simulink model "zynqRadioWLAN80211BeaconRxFPGAAD9361AD9364RetargetSL"  (R2016a)
settings: Solver=FixedStepDiscrete  SolverMode=SingleTasking  StartTime=0.0  StopTime=inf  RelTol=1e-3
PreLoadFcn:
  | load('commwlan80211BusTypes')
  | openMPDUGUI = true;
PostLoadFcn:
  | zynqRadioWLAN80211BeaconRxFPGAAD9361AD9364SL_params('init')
  | zynqRadioWLAN80211BeaconRxFPGAAD9361AD9364SL_params('retarget_scope')
InitFcn:
  | load('commwlan80211BusTypes')
  | openMPDUGUI = true;
  | mpduFigPos= [ 100 100 400 500];
model workspace: external: MAT-File (data not in the file)
undefined symbols (not defined in the file or in its folder): F, p80211
libraries: commutil2 x3, hdlsllib x3, commwlan80211BeaconLib x2, commdigbbndpm3 x1, commsequence2 x1, simulink x1, commcrc2 x1, sdrzblksprivate x1, zc706fmc234_lib x1
CloseFcn:
  | clear BeaconFrameBodyType BeaconMPDUType CapabilityType FrameCtrlType InfoElementType MPDUHeaderType p80211 commwlan80211TxFilt rcvd openMPDUGUI mpduFigPos p80211hdl Hd
  | hFig = findall(0, 'Type', 'figure', 'Name', '802.11 Beacon Frame');
  | if ishghandle(hFig)
  | close(hFig);
  | end
  | clear hFig
  | if (exist('ans')==1) && (iscell(ans) && (numel(ans) == 0))
  | clear ans
  | end
Description:
  | IEEE 802.11 WLAN Beacon Frame Receiver for Captured Data
  | 
  | This example shows how to process a captured beacon frame and display the
  | frame information.
settings Model: ModifiedByFormat=The MathWorks Inc.  SimulationMode=accelerator  ExtModeTrigDuration=100  Creator=The MathWorks, Inc.  LastModifiedBy=The MathWorks Inc.
settings DataIOCC: LimitDataPoints=on  SaveFormat=Array  SaveOutput=off  SignalLogging=off  DSMLogging=off  StateSaveName=tmp_raccel_xout
settings OptimizationCC: BlockReduction=off  ConditionallyExecuteInputs=off  DefaultParameterBehavior=Inlined  InlineInvariantSignals=on  ExpressionDepthLimit=2147483647  EfficientMapNaN2IntZero=off
settings DebuggingCC: ReadBeforeWriteMsg=DisableAll  WriteAfterWriteMsg=DisableAll  WriteAfterReadMsg=DisableAll  AlgebraicLoopMsg=error  UnderspecifiedInitializationDetection=Classic  MergeDetectMultiDrivingBlocksExec=none  SolverPrmCheckMsg=warning  InheritedTsInSrcMsg=none  SingleTaskRateTransMsg=error  IntegerOverflowMsg=none  ParameterDowncastMsg=none  ParameterOverflowMsg=none  ParameterPrecisionLossMsg=none  ParameterTunabilityLossMsg=none  UniqueDataStoreMsg=error  AllowSymbolicDim=off  ModelReferenceDataLoggingMessage=none  StateNameClashWarn=warning  IntegerSaturationMsg=none
settings HardwareCC: ProdBitPerPointer=32  ProdLargestAtomicFloat=None  ProdIntDivRoundTo=Undefined  ProdEndianess=Unspecified  ProdWordSize=32  ProdHWDeviceType=ASIC/FPGA->ASIC/FPGA  TargetBitPerPointer=64  TargetLongLongMode=on  TargetIntDivRoundTo=Zero  TargetEndianess=LittleEndian  TargetWordSize=64  TargetHWDeviceType=MATLAB Host  ProdEqTarget=off
settings ModelReferenceCC: PropagateSignalLabelsOutOfModel=off
settings RTWCC: SystemTargetFile=raccel.tlc  TemplateMakefile=raccel_default_tmf  RTWVerbose=off  RTWUseSimCustomCode=on
settings CodeAppCC: GenerateComments=off  MaxIdLength=128  MangleLength=10  SimulinkBlockComments=off
settings RaccelTargetCC: ERTMultiwordTypeDef=System defined  ERTMultiwordLength=256  ParMdlRefBuildCompliant=off  GeneratePreprocessorConditionals=Disable all  ERTFirstTimeCompliant=off  MultiInstanceERTCode=off  ENABLE_SLEXEC_SSBRIDGE=0  RTWCAPISignals=off  RTWCAPIParams=off
settings ConfigComp: CovModelRefEnable=Off  CovSFcnEnable=off

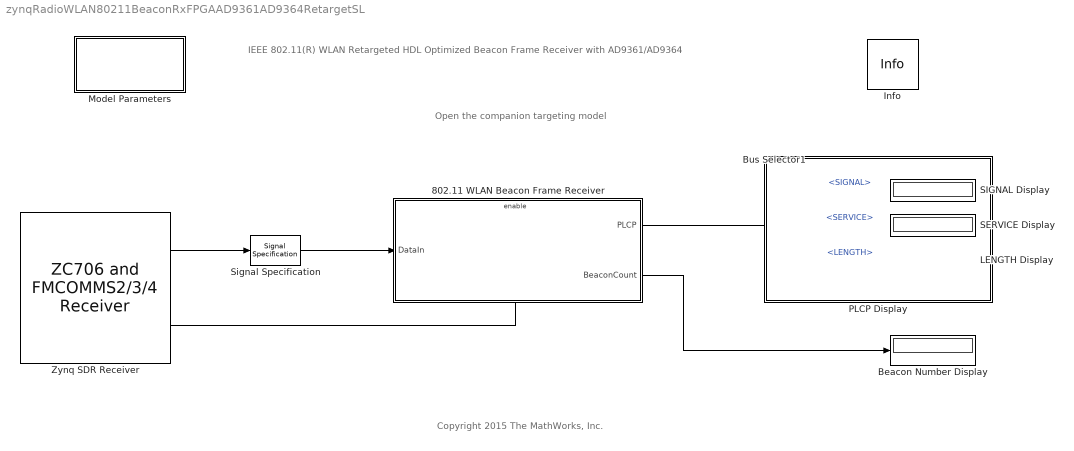
== system zynqRadioWLAN80211BeaconRxFPGAAD9361AD9364RetargetSL ==
  note: IEEE 802.11(R) WLAN
      | Retargeted HDL Optimized Beacon Frame Receiver with AD9361/AD9364
  note: Copyright 2015 The MathWorks, Inc.
  note: Open the companion targeting model
  802.11 WLAN Beacon Frame Receiver : Subsystem
  Beacon Number Display : Display
  Bus Selector1 : BusSelector  OutputSignals=SIGNAL,SERVICE,LENGTH
  Info : sdrzblksprivate/Info  SystemSampleTime=-1
  LENGTH Display : Display
  Model Parameters : Subsystem  mask(Model Parameters){chanNum=1, rfGain=30, rfFreqOffset=0}
      mask prompts: chanNum "Channel number"; rfGain "RF board gain:"; rfFreqOffset "RF center frequency offset:"
      mask help:
      | Choose 802.11 receiver parameters.
      |
      | You can select channel number for the 802.11 signals. You can set the AGC parameters and samples per chip used in the receiver. You can also set the synchronization threshold value to determine the correlation threshold used to declare the presence of an 802.11 packet.
      mask init:
      | zynqRadioWLAN80211BeaconRxFPGAAD9361AD9364SL_params('init', ...
      |     'ChannelNumber',   chanNum, ...
      |     'RadioGain',       rfGain, ...
      |     'RadioFreqOffset', rfFreqOffset ...
      |     );
      mask TypeOptions chanNum: 1 | 2 | 3 | 4 | 5 | 6 | 7 | 8 | 9 | 10 | 11
      mask Display: disp('Model\nParameters')
  PLCP Display : Subsystem
      mask Display: disp('')
  SERVICE Display : Display
      settings: Format=hex (Stored Integer)
  SIGNAL Display : Display
      settings: Format=hex (Stored Integer)
  Signal Specification : SignalSpecification  SampleTime=p80211.RadioFrameLength/p80211.RadioBasebandRate
  Zynq SDR Receiver : zc706fmc234_lib/ZC706 and  FMCOMMS2//3//4  Receiver  IPAddress=192.168.3.2  CenterFrequencySource=Dialog  CenterFrequency=2.412e9+(p80211.ChannelNumber-1)*5e6+p80211.RadioFreqOffset  GainSource=Dialog  Gain=p80211.RadioGain  ChannelMapping=1  BasebandSampleRate=p80211.RadioBasebandRate  EnableBurstMode=on  NumFramesInBurst=p80211.RadioNumFramesInBurst  OutputDataType=int16  SamplesPerFrame=p80211.RadioFrameLength  LostSamplesOutputPort=off  RSSIOutputPort=off  DMATimeoutValue=1  blockMode=Normal  EnableQuadratureTracking=on  EnableRFDCTracking=on  EnableBasebandDCTracking=on  BypassUserLogic=off  ShowAdvancedProperties=on  ShowInternalProperties=off  subDeviceList=zynqReceiver  sdrExecutionMode=HW  dataUDPPort=-1  ctrlUDPPort=-1  SourceSelect=RF data  SourceConfiguration1=1023  FIRCoefficientSize=[ 128; 128 ]  FIRCoefficients=[ 111, -87, 147, -127, -18, -286, -312, -555, -601, -722, -642, -555, -303, -66, 221, 393, 488, 403, 219, -74, -343, -550, -582, -450, -146, 221, 569, 759, 735, 463, 20, -487, -885, -1048, -883, -418, 243, 897, 1340, 1394, 1002, 228, -715, -1549, -1980, -1819, -1028, 217, 1583, 2635, 2980, 2377, 853, -1275, -3435, -4926, -5080, -3454, 40, 5065, 10903, 16581, 21085, 23573, 23573, 21085, 16581, 10903, 5065, 40, -3454, -5080, -4926, -3435, -1275, 853, 2377, 2980, 2635, 1583, 217, -1028, -1819, -1980, -1549, -715, 228, 1002, 1394, 1340, 897, 243, -418, -883, -1048, -885, -487, 20, 463, 735, 759, 569, 221, -146, -450, -582, -550, -343, -74, 219, 403, 488, 393, 221, -66, -303, -555, -642, -722, -601, -555, -312, -286, -18, -127, 147, -87, 111; 382, -200, 711, -41, 645, 36, 346, -194, -119, -543, -472, -646, -404, -312, 45, 197, 413, 346, 241, -93, -373, -680, -755, -689, -356, 51, 515, 795, 870, 609, 136, -488, -1009, -1303, -1191, -712, 69, 885, 1516, 1692, 1336, 468, -662, -1740, -2378, -2329, -1494, -55, 1620, 2995, 3584, 3045, 1368, -1121, -3755, -5708, -6156, -4542, -710, 4969, 11669, 18243, 23486, 26391, 26391, 23486, 18243, 11669, 4969, -710, -4542, -6156, -5708, -3755, -1121, 1368, 3045, 3584, 2995, 1620, -55, -1494, -2329, -2378, -1740, -662, 468, 1336, 1692, 1516, 885, 69, -712, -1191, -1303, -1009, -488, 136, 609, 870, 795, 515, 51, -356, -689, -755, -680, -373, -93, 241, 346, 413, 197, 45, -312, -404, -646, -472, -543, -119, -194, 346, 36, 645, -41, 711, -200, 382 ]  FIRGain=[ 0; -12 ]  FIRDecimInterpFactor=[ 4; 4 ]  AnalogFilterCutoff=[ 2560000; 2560000 ]  FilterPathRates=[ 737280000, 184320000, 61440000, 30720000, 15360000, 3840000; 737280000, 184320000, 61440000, 30720000, 15360000, 3840000 ]  FilterDesignTypeForTx=DefaultFilterFromOther  FilterDesignTypeForRx=DefaultFilter  BISTLoopbackConfig=No Loopback  BISTPRBSMode=PRBS Disable  BISTToneMode=Tone Disable  BISTToneFrequency=F/32  BISTToneLevel=-6  BISTChannelMask=0  DataIsComplex=on  SimulateUsing=Code generation
  wires:
  802.11 WLAN Beacon Frame Receiver/1(PLCP) -> Bus Selector1/1
  Bus Selector1/3 -> LENGTH Display/1  "<LENGTH>"
  Bus Selector1/1 -> SIGNAL Display/1  "<SIGNAL>"
  Bus Selector1/2 -> SERVICE Display/1  "<SERVICE>"
  Zynq SDR Receiver/1 -> Signal Specification/1
  Zynq SDR Receiver/2 -> 802.11 WLAN Beacon Frame Receiver/Enable
  Signal Specification/1 -> 802.11 WLAN Beacon Frame Receiver/1(DataIn)
  802.11 WLAN Beacon Frame Receiver/2(BeaconCount) -> Beacon Number Display/1

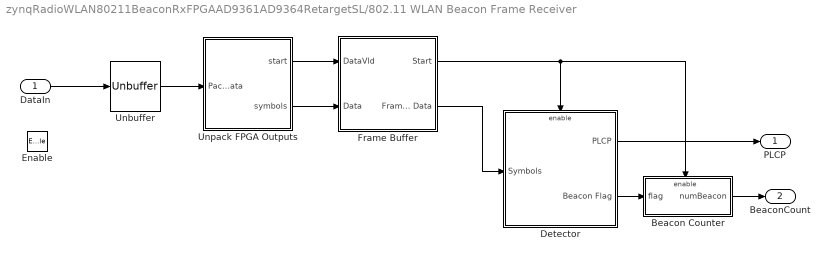
== system zynqRadioWLAN80211BeaconRxFPGAAD9361AD9364RetargetSL/802.11 WLAN Beacon Frame Receiver ==
  DataIn : Inport
  Enable : EnablePort
  Beacon Counter : Subsystem
  Detector : Subsystem
      settings: CloseFcn=clear BeaconFrameBodyType rcvd
  Frame Buffer : Subsystem
  Unbuffer : Unbuffer  SampleBasedProcessing=Same as frame based
  Unpack FPGA Outputs : Subsystem
  PLCP : Outport
  BeaconCount : Outport  Port=2
  wires:
  Frame Buffer/1(Start) -> Detector/Enable, Beacon Counter/Enable
  Frame Buffer/2(Framed Data) -> Detector/1(Symbols)
  Beacon Counter/1(numBeacon) -> BeaconCount/1
  DataIn/1 -> Unbuffer/1
  Detector/1(PLCP) -> PLCP/1
  Detector/2(Beacon Flag) -> Beacon Counter/1(flag)
  Unbuffer/1 -> Unpack FPGA Outputs/1(PackedData)
  Unpack FPGA Outputs/1(start) -> Frame Buffer/1(DataVld)
  Unpack FPGA Outputs/2(symbols) -> Frame Buffer/2(Data)

== system zynqRadioWLAN80211BeaconRxFPGAAD9361AD9364RetargetSL/Model Parameters ==

== system zynqRadioWLAN80211BeaconRxFPGAAD9361AD9364RetargetSL/PLCP Display ==

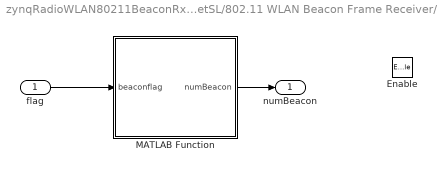
== system zynqRadioWLAN80211BeaconRxFPGAAD9361AD9364RetargetSL/802.11 WLAN Beacon Frame Receiver/Beacon Counter ==
  flag : Inport
  Enable : EnablePort
  MATLAB Function : MATLAB Function  TreatAsAtomicUnit=on
  numBeacon : Outport
  wires:
  MATLAB Function/1(numBeacon) -> numBeacon/1
  flag/1 -> MATLAB Function/1(beaconflag)

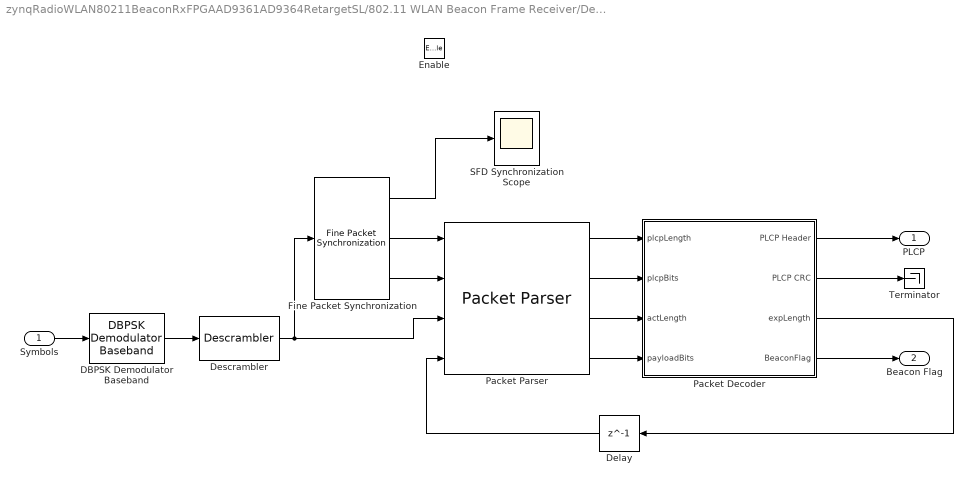
== system zynqRadioWLAN80211BeaconRxFPGAAD9361AD9364RetargetSL/802.11 WLAN Beacon Frame Receiver/Detector ==
  Symbols : Inport
  Enable : EnablePort  StatesWhenEnabling=reset  PropagateVarSize=During execution
  DBPSK Demodulator Baseband : commdigbbndpm3/DBPSK Demodulator Baseband  Ph=0  outDtype=uint32
  Delay : Delay  DelayLength=1  InitialCondition=0  InputProcessing=Columns as channels (frame based)
  Descrambler : commsequence2/Descrambler  M=2  poly=p80211.ScramblerPolynomial  iniStaSource=Dialog Parameter  ini_sta=[0 0 0 0 0 0 0]  resetViaPort=off
  Fine Packet Synchronization : commwlan80211BeaconLib/Fine Packet Synchronization
  Packet Decoder : Subsystem
  Packet Parser : commwlan80211BeaconLib/Packet Parser
  SFD Synchronization Scope : Scope
      settings: Priority=10
  Terminator : Terminator
  PLCP : Outport
  Beacon Flag : Outport  Port=2  InitialOutput=1
  wires:
  Fine Packet Synchronization/1 -> SFD Synchronization Scope/1
  DBPSK Demodulator Baseband/1 -> Descrambler/1
  Symbols/1 -> DBPSK Demodulator Baseband/1
  Descrambler/1 -> Fine Packet Synchronization/1, Packet Parser/3
  Fine Packet Synchronization/2 -> Packet Parser/1
  Fine Packet Synchronization/3 -> Packet Parser/2
  Delay/1 -> Packet Parser/4
  Packet Parser/2 -> Packet Decoder/2(plcpBits)
  Packet Parser/3 -> Packet Decoder/3(actLength)
  Packet Parser/4 -> Packet Decoder/4(payloadBits)
  Packet Decoder/1(PLCP Header) -> PLCP/1
  Packet Parser/1 -> Packet Decoder/1(plcpLength)
  Packet Decoder/2(PLCP CRC) -> Terminator/1
  Packet Decoder/3(expLength) -> Delay/1
  Packet Decoder/4(BeaconFlag) -> Beacon Flag/1

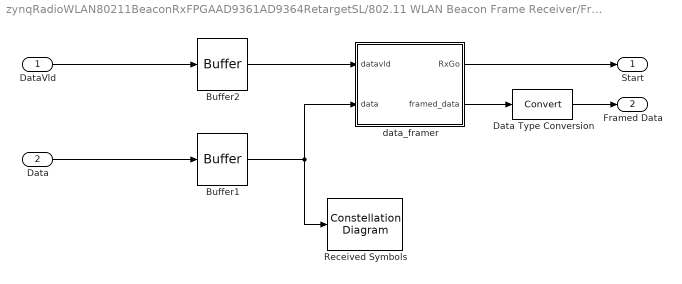
== system zynqRadioWLAN80211BeaconRxFPGAAD9361AD9364RetargetSL/802.11 WLAN Beacon Frame Receiver/Frame Buffer ==
  DataVld : Inport
  Data : Inport  Port=2
  Buffer1 : Buffer  N=128  TreatMby1Signals=One channel  OutputFrames=off
  Buffer2 : Buffer  N=128  TreatMby1Signals=One channel  OutputFrames=off
  Data Type Conversion : DataTypeConversion
  Received Symbols : ConstellationDiagram  Tag=ScatterPlot  Priority=2
  data_framer : MATLAB Function  TreatAsAtomicUnit=on
  Start : Outport
  Framed Data : Outport  Port=2
  wires:
  Data Type Conversion/1 -> Framed Data/1
  data_framer/2(framed_data) -> Data Type Conversion/1
  data_framer/1(RxGo) -> Start/1
  Buffer1/1 -> data_framer/2(data), Received Symbols/1
  DataVld/1 -> Buffer2/1
  Data/1 -> Buffer1/1
  Buffer2/1 -> data_framer/1(datavld)

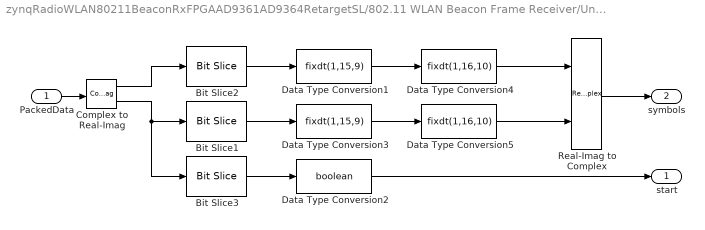
== system zynqRadioWLAN80211BeaconRxFPGAAD9361AD9364RetargetSL/802.11 WLAN Beacon Frame Receiver/Unpack FPGA Outputs ==
  PackedData : Inport
  Bit Slice1 : hdlsllib/HDL Operations/Bit Slice  lidx=15  ridx=1
  Bit Slice2 : hdlsllib/HDL Operations/Bit Slice  lidx=15  ridx=1
  Bit Slice3 : hdlsllib/HDL Operations/Bit Slice  lidx=0  ridx=0
  Complex to Real-Imag : ComplexToRealImag
  Data Type Conversion1 : DataTypeConversion  OutDataTypeStr=fixdt(1,15,9)  ConvertRealWorld=Stored Integer (SI)
  Data Type Conversion2 : DataTypeConversion  OutDataTypeStr=boolean
  Data Type Conversion3 : DataTypeConversion  OutDataTypeStr=fixdt(1,15,9)  ConvertRealWorld=Stored Integer (SI)
  Data Type Conversion4 : DataTypeConversion  OutDataTypeStr=fixdt(1,16,10)
  Data Type Conversion5 : DataTypeConversion  OutDataTypeStr=fixdt(1,16,10)
  Real-Imag to Complex : RealImagToComplex
  start : Outport
  symbols : Outport  Port=2
  wires:
  PackedData/1 -> Complex to Real-Imag/1
  Real-Imag to Complex/1 -> symbols/1
  Complex to Real-Imag/1 -> Bit Slice2/1
  Complex to Real-Imag/2 -> Bit Slice3/1, Bit Slice1/1
  Bit Slice3/1 -> Data Type Conversion2/1
  Data Type Conversion2/1 -> start/1
  Bit Slice2/1 -> Data Type Conversion1/1
  Bit Slice1/1 -> Data Type Conversion3/1
  Data Type Conversion1/1 -> Data Type Conversion4/1
  Data Type Conversion4/1 -> Real-Imag to Complex/1
  Data Type Conversion3/1 -> Data Type Conversion5/1
  Data Type Conversion5/1 -> Real-Imag to Complex/2

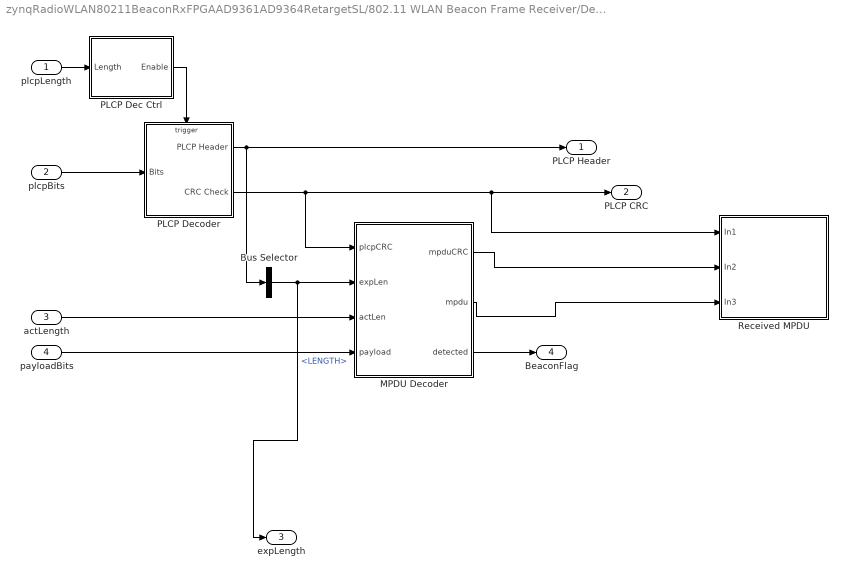
== system zynqRadioWLAN80211BeaconRxFPGAAD9361AD9364RetargetSL/802.11 WLAN Beacon Frame Receiver/Detector/Packet Decoder ==
  plcpLength : Inport
  plcpBits : Inport  Port=2
  actLength : Inport  Port=3
  payloadBits : Inport  Port=4
  Bus Selector : BusSelector  OutputSignals=LENGTH
  MPDU Decoder : MATLAB Function  TreatAsAtomicUnit=on
  PLCP Dec Ctrl : Subsystem
  PLCP Decoder : Subsystem
  Received MPDU : Subsystem  mask(MPDU GUI){OpenScopeAtSimStart=openMPDUGUI, figPosition=mpduFigPos}
      mask prompts: OpenScopeAtSimStart "Open GUI at start of simulation"; figPosition "Position"
      mask help: Display contents of the MPDU.
      mask Display: disp('MPDU GUI')
  PLCP Header : Outport
  PLCP CRC : Outport  Port=2
  expLength : Outport  Port=3
  BeaconFlag : Outport  Port=4
  wires:
  PLCP Dec Ctrl/1(Enable) -> PLCP Decoder/Trigger
  Bus Selector/1 -> MPDU Decoder/2(expLen), expLength/1  "<LENGTH>"
  PLCP Decoder/1(PLCP Header) -> Bus Selector/1, PLCP Header/1
  plcpLength/1 -> PLCP Dec Ctrl/1(Length)
  plcpBits/1 -> PLCP Decoder/1(Bits)
  actLength/1 -> MPDU Decoder/3(actLen)
  payloadBits/1 -> MPDU Decoder/4(payload)
  MPDU Decoder/1(mpduCRC) -> Received MPDU/2(In2)
  MPDU Decoder/2(mpdu) -> Received MPDU/3(In3)
  PLCP Decoder/2(CRC Check) -> MPDU Decoder/1(plcpCRC), Received MPDU/1(In1), PLCP CRC/1
  MPDU Decoder/3(detected) -> BeaconFlag/1

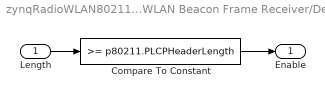
== system zynqRadioWLAN80211BeaconRxFPGAAD9361AD9364RetargetSL/802.11 WLAN Beacon Frame Receiver/Detector/Packet Decoder/PLCP Dec Ctrl ==
  Length : Inport
  Compare To Constant : simulink/Logic and Bit Operations/Compare To Constant  relop=>=  const=p80211.PLCPHeaderLength  OutDataTypeStr=uint8
  Enable : Outport
  wires:
  Length/1 -> Compare To Constant/1
  Compare To Constant/1 -> Enable/1

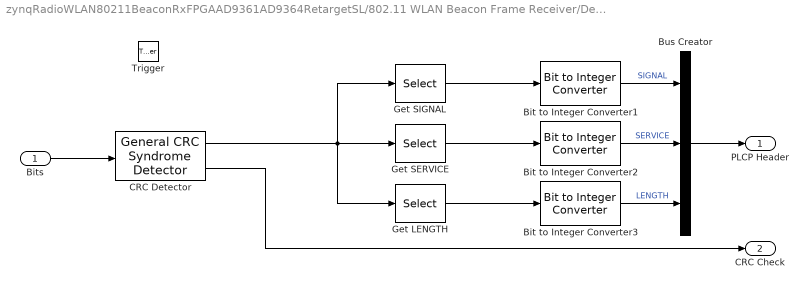
== system zynqRadioWLAN80211BeaconRxFPGAAD9361AD9364RetargetSL/802.11 WLAN Beacon Frame Receiver/Detector/Packet Decoder/PLCP Decoder ==
  Bits : Inport
  Trigger : TriggerPort  VariantControl=Variant  PortDimensions=1
  Bit to Integer Converter1 : commutil2/Bit to Integer Converter  nbits=8  bitOrder=LSB first  signedOutputValues=Unsigned  outDtype=Inherit via internal rule  outDtypeSigned=Inherit via internal rule
  Bit to Integer Converter2 : commutil2/Bit to Integer Converter  nbits=8  bitOrder=LSB first  signedOutputValues=Unsigned  outDtype=Inherit via internal rule  outDtypeSigned=Inherit via internal rule
  Bit to Integer Converter3 : commutil2/Bit to Integer Converter  nbits=16  bitOrder=LSB first  signedOutputValues=Unsigned  outDtype=uint16  outDtypeSigned=Inherit via internal rule
  Bus Creator : BusCreator  Inputs=3
  CRC Detector : commcrc2/General CRC Syndrome Detector  genPoly=[1 0 0 0 1 0 0 0 0 0 0 1 0 0 0 0 1]  iniStates=1  directMethod=on  reflectInputBytes=off  reflectChecksums=off  finalXOR=1  numChecksums=1
  Get LENGTH : Selector  InputPortWidth=32  IndexOptions=Index vector (dialog)  Indices=17:32  OutputSizes=1
  Get SERVICE : Selector  InputPortWidth=32  IndexOptions=Index vector (dialog)  Indices=9:16  OutputSizes=1
  Get SIGNAL : Selector  InputPortWidth=32  IndexOptions=Index vector (dialog)  Indices=1:8  OutputSizes=1
  PLCP Header : Outport
  CRC Check : Outport  Port=2
  wires:
  Bus Creator/1 -> PLCP Header/1
  Bit to Integer Converter3/1 -> Bus Creator/3  "LENGTH"
  Bits/1 -> CRC Detector/1
  Bit to Integer Converter2/1 -> Bus Creator/2  "SERVICE"
  Bit to Integer Converter1/1 -> Bus Creator/1  "SIGNAL"
  Get LENGTH/1 -> Bit to Integer Converter3/1
  Get SERVICE/1 -> Bit to Integer Converter2/1
  Get SIGNAL/1 -> Bit to Integer Converter1/1
  CRC Detector/1 -> Get SIGNAL/1, Get SERVICE/1, Get LENGTH/1
  CRC Detector/2 -> CRC Check/1

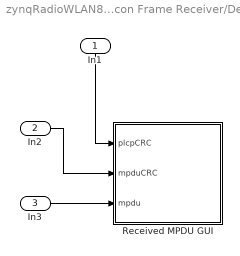
== system zynqRadioWLAN80211BeaconRxFPGAAD9361AD9364RetargetSL/802.11 WLAN Beacon Frame Receiver/Detector/Packet Decoder/Received MPDU ==
  In1 : Inport
  In2 : Inport  Port=2
  In3 : Inport  Port=3
  Received MPDU GUI : MATLAB Function  TreatAsAtomicUnit=on
  wires:
  In3/1 -> Received MPDU GUI/3(mpdu)
  In2/1 -> Received MPDU GUI/2(mpduCRC)
  In1/1 -> Received MPDU GUI/1(plcpCRC)

== matlab function zynqRadioWLAN80211BeaconRxFPGAAD9361AD9364RetargetSL/802.11 WLAN Beacon Frame Receiver/Detector/Packet Decoder/MPDU Decoder ==
  data: mpduCRC output; plcpCRC input boolean size=1; expLen input size=1; actLen input; payload input; mpdu output Bus: BeaconMPDUType size=[1 1]; detected output
function [mpduCRC, mpdu,detected] = mpduDec(plcpCRC, expLen, actLen, payload)
%#codegen

coder.extrinsic('warning')

persistent hCRC firstTime lastMPDU lastMpduCRC 

% Frame check sequence (FCS)
if isempty(hCRC)
  hCRC = comm.CRCDetector([32 26 23 22 16 12 11 10 8 7 5 4 2 1 0], ...
    'InitialConditions', 1, ...
    'DirectMethod',      true, ...
    'FinalXOR',          1);
  firstTime = true;
  lastMPDU.Header = parseMPDUHeader(zeros(64,1), 1);
  lastMPDU.FrameBody = unknownMPDU();
  lastMpduCRC = true;  % CRC is not zero
 
end

% If the CRC for the header decodes correctly (i.e. CRC flag is 0) and the
% received MPDU payload length is greater than or equal to the expected
% length, then turn on the MPDU decoder
detected = false;
if ~plcpCRC && (expLen > 0) && (actLen >= expLen) && (expLen >= 32) ...
    && firstTime
  % Compute CRC based on IEEE Std 802.11(TM)-2007 section 7.1.3.7.
  frameCRC = payload(1:expLen);
  [frame, mpduCRC] = step(hCRC, frameCRC);
  
  [mpdu.Header, mpduHeaderLen] = parseMPDUHeader(frame, mpduCRC);

  
  if (mpduCRC == 1) || ((mpdu.Header.FrameCtrl.Type ~= 0) ...
      || (mpdu.Header.FrameCtrl.Subtype ~= 8))
    mpdu.FrameBody = unknownMPDU();
   else
    mpdu.FrameBody = parseBeaconMPDU(frame(mpduHeaderLen+1:end, 1), mpduCRC);
    detected = true;
  end
  
  lastMPDU = mpdu;
  lastMpduCRC = mpduCRC;
  firstTime = false;
else
  mpdu = lastMPDU;
  mpduCRC = lastMpduCRC;
end

end

function [mpduHeader, len] = parseMPDUHeader(frame, mpduCRC)
% Based on IEEE Std 802.11-2007 chapter 7.

mpduHeader.FrameCtrl       = parseFrameControl(frame(1:16,1), mpduCRC);
mpduHeader.DurationID      = zeros(1,2,'uint8');
mpduHeader.Address1        = zeros(1,6,'uint8');
mpduHeader.Address2        = zeros(1,6,'uint8');
mpduHeader.Address3        = zeros(1,6,'uint8');
mpduHeader.SequenceControl = zeros(1,2,'uint8');
mpduHeader.Address4        = zeros(1,6,'uint8');
len = (2+6+6+6+2+6)*8 + 16;

if (mpduCRC == 0)
  p = 1;
  mpduHeader.FrameCtrl       = parseFrameControl(frame(p:p+15,1), mpduCRC);
  p = p+16;
  mpduHeader.DurationID      = bit2Octet(frame(p:p+15,1),2);
  p = p+16;
  mpduHeader.Address1        = bit2Octet(frame(p:p+47,1),6);
  p = p+48;
  
  isManagementFrame = (mpduHeader.FrameCtrl.Type == 0);
  isControlFrame = (mpduHeader.FrameCtrl.Type == 1);
  isDataFrame = (mpduHeader.FrameCtrl.Type == 2);
  isCTSFrame = isControlFrame && (mpduHeader.FrameCtrl.Subtype == 12);
  isACKFrame = isControlFrame && (mpduHeader.FrameCtrl.Subtype == 13);
  
  if ~(isCTSFrame || isACKFrame)
    mpduHeader.Address2        = bit2Octet(frame(p:p+47,1),6);
    p = p+48;
  end
  if isManagementFrame 
    mpduHeader.Address3        = bit2Octet(frame(p:p+47,1),6);
    p = p+48;
  end
  if ~isControlFrame
    mpduHeader.SequenceControl = bit2Octet(frame(p:p+15,1),2);
    p = p+16;
  end
  if isDataFrame
    mpduHeader.Address4        = bit2Octet(frame(p:p+47,1),6);
    p = p+48;
  end
  len = p-1;
end
end

function frameCtrl = parseFrameControl(fcBits, mpduCRC)
if (mpduCRC == 0)
  frameCtrl.ProtocolVersion = uint8(bi2de(fcBits(1:2,1)'));
  frameCtrl.Type            = uint8(bi2de(fcBits(3:4,1)'));
  frameCtrl.Subtype         = uint8(bi2de(fcBits(5:8,1)'));
  frameCtrl.ToDS            = uint8(bi2de(fcBits(9,1)'));
  frameCtrl.FromDS          = uint8(bi2de(fcBits(10,1)'));
  frameCtrl.MoreFragments   = uint8(bi2de(fcBits(11,1)'));
  frameCtrl.Retry           = uint8(bi2de(fcBits(12,1)'));
  frameCtrl.PowerManagement = uint8(bi2de(fcBits(13,1)'));
  frameCtrl.MoreData        = uint8(bi2de(fcBits(14,1)'));
  frameCtrl.ProtectedFrame  = uint8(bi2de(fcBits(15,1)'));
  frameCtrl.Order           = uint8(bi2de(fcBits(16,1)'));
else
  frameCtrl.ProtocolVersion = uint8(0);
  frameCtrl.Type            = uint8(0);
  frameCtrl.Subtype         = uint8(0);
  frameCtrl.ToDS            = uint8(0);
  frameCtrl.FromDS          = uint8(0);
  frameCtrl.MoreFragments   = uint8(0);
  frameCtrl.Retry           = uint8(0);
  frameCtrl.PowerManagement = uint8(0);
  frameCtrl.MoreData        = uint8(0);
  frameCtrl.ProtectedFrame  = uint8(0);
  frameCtrl.Order           = uint8(0);
end
end

function frameBody = parseBeaconMPDU(frame, mpduCRC)
if (mpduCRC == 0)
  bitCount = uint32(1);
  frameBody.TimeStamp      = bit2Octet(frame(bitCount:bitCount+63,1),8);
  bitCount = bitCount + 64;
  frameBody.BeaconInterval = bit2Octet(frame(bitCount:bitCount+15,1),2);
  bitCount = bitCount + 16;
  frameBody.Capability     = parseCapabilities(frame(81:96), mpduCRC);
  bitCount = bitCount + 16;
else
  frameBody.TimeStamp      = zeros(1,8,'uint8');
  frameBody.BeaconInterval = zeros(1,2,'uint8');
  frameBody.Capability     = parseCapabilities(frame(81:96), mpduCRC);
  bitCount = uint32(97);
end

frameLength = length(frame);

frameBody.NumInfoElements = uint8(0);
macElementStruct = struct('ID', uint8(255), ...
  'Length', uint8(0), ...
  'Value', zeros(1,257,'uint8'));
frameBody.InfoElements = repmat(macElementStruct, 1, 60);

if (mpduCRC == 0)
  while bitCount < frameLength
    frameBody.NumInfoElements = frameBody.NumInfoElements + 1;
    frameBody.InfoElements(frameBody.NumInfoElements).ID = ...
      bit2Octet(frame(bitCount:bitCount+7,1), 1);
    bitCount = bitCount + 8;
    elemLength = bit2Octet(frame(bitCount:bitCount+7,1), 1);
    frameBody.InfoElements(frameBody.NumInfoElements).Length = elemLength;
    bitCount = bitCount + 8;
    for p=1:elemLength
      frameBody.InfoElements(frameBody.NumInfoElements).Value(p) = ...
        bit2Octet(frame(bitCount:bitCount+7),1);
      bitCount = bitCount+8;
    end
  end
end
end

function capability = parseCapabilities(frame, mpduCRC)
if (mpduCRC == 0)
  capability.ESS                = frame(1,1);
  capability.IBSS               = frame(2,1);
  capability.CFPollable         = frame(3,1);
  capability.CFPollRequest      = frame(4,1);
  capability.Privacy            = frame(5,1);
  capability.ShortPreamble      = frame(6,1);
  capability.PBCC               = frame(7,1);
  capability.ChannelAgility     = frame(8,1);
  capability.SpectrumManagement = frame(9,1);
  capability.QoS                = frame(10,1);
  capability.ShortSlotTime      = frame(11,1);
  capability.APSD               = frame(12,1);
  capability.Reserved           = frame(13,1);
  capability.DSSOFDM            = frame(14,1);
  capability.DelayedBlockAck    = frame(15,1);
  capability.ImmediateBlockAck  = frame(16,1);
else
  capability.ESS                = false;
  capability.IBSS               = false;
  capability.CFPollable         = false;
  capability.CFPollRequest      = false;
  capability.Privacy            = false;
  capability.ShortPreamble      = false;
  capability.PBCC               = false;
  capability.ChannelAgility     = false;
  capability.SpectrumManagement = false;
  capability.QoS                = false;
  capability.ShortSlotTime      = false;
  capability.APSD               = false;
  capability.Reserved           = false;
  capability.DSSOFDM            = false;
  capability.DelayedBlockAck    = false;
  capability.ImmediateBlockAck  = false;
end
end

function frameBody = unknownMPDU()
frameBody.TimeStamp      = zeros(1,8,'uint8');
frameBody.BeaconInterval = zeros(1,2,'uint8');
frameBody.Capability     = parseCapabilities(zeros(16,1), 1);

frameBody.NumInfoElements = uint8(0);
macElementStruct = struct('ID', uint8(255), ...
  'Length', uint8(0), ...
  'Value', zeros(1,257,'uint8'));
frameBody.InfoElements = repmat(macElementStruct, 1, 60);
end

function octets = bit2Octet(bits,numOctets)
octets = zeros(1, numOctets, 'uint8');
for p=1:numOctets
  octets(1,p) = (bits((p-1)*8+1:p*8)')*2.^(0:7)';
end
end

== matlab function zynqRadioWLAN80211BeaconRxFPGAAD9361AD9364RetargetSL/802.11 WLAN Beacon Frame Receiver/Detector/Packet Decoder/Received MPDU/Received MPDU GUI ==
  data: plcpCRC input; mpduCRC input; mpdu input; OpenScopeAtSimStart parameter size=[1 1]; figPosition parameter
function mpduGUI(plcpCRC, mpduCRC, mpdu, OpenScopeAtSimStart, figPosition)
%#codegen

persistent resetGUI

if isempty(resetGUI)
  resetGUI = true;
end

coder.extrinsic('receivedFullMPDUGUI')

receivedFullMPDUGUI(mpdu.Header, mpdu.FrameBody, plcpCRC, mpduCRC, ...
  resetGUI, OpenScopeAtSimStart, figPosition);

resetGUI = false;

== matlab function zynqRadioWLAN80211BeaconRxFPGAAD9361AD9364RetargetSL/802.11 WLAN Beacon Frame Receiver/Beacon Counter/MATLAB Function ==
  data: numBeacon output; beaconflag input
function numBeacon   = fcn(beaconflag)


%#codegen


persistent   beaconcnt

if isempty (beaconcnt)
    beaconcnt = 0;
    
end

if beaconflag
    
    beaconcnt = beaconcnt+1;
    
end

numBeacon = beaconcnt;

== matlab function zynqRadioWLAN80211BeaconRxFPGAAD9361AD9364RetargetSL/802.11 WLAN Beacon Frame Receiver/Frame Buffer/data_framer ==
  data: datavld input; data input; RxGo output; p80211 parameter; framed_data output
function [RxGo, framed_data] = dataframer(datavld, data, p80211)
%#codegen

persistent  gooddata_from_prev length_prev_good_data


if isempty(gooddata_from_prev)
    gooddata_from_prev = complex(zeros(128,1));
    length_prev_good_data = 0;
end

if any(datavld) % there is some valid data
    % get the valid data from this frame and append it with the previous
    % stored one, if any
    gooddata_current = data(logical(datavld));
    % append with prev good data
    data_tmp = [gooddata_from_prev(1:length_prev_good_data);gooddata_current];
    if length(data_tmp) > 128
        framed_data = data_tmp(1:128);
        RxGo = 1;
        gooddata_length_athand = length(data_tmp);
        datalen_fornext = gooddata_length_athand -128;
        gooddata_from_prev(1:datalen_fornext) = data_tmp(129:129+datalen_fornext-1);
        length_prev_good_data = datalen_fornext;
    elseif length(data_tmp) == 128 
        framed_data = data_tmp(1:128);
        RxGo = 1;
        gooddata_from_prev =  complex(zeros(128,1));
        length_prev_good_data = 0;
    else % less than 128
        gooddata_length_athand = length(data_tmp);
        datalen_fornext = gooddata_length_athand;      
        gooddata_from_prev(1:gooddata_length_athand) = data_tmp(1:gooddata_length_athand);
        length_prev_good_data = datalen_fornext;
        framed_data = data; % garbage
        RxGo = 0;
    end
    
else % none of the data is valid
    RxGo = 0;
    framed_data = data; %just send the data through
    gooddata_from_prev = complex(zeros(128,1));
    length_prev_good_data = 0;
end
